simulink model "Ejercicio4_23_03_17"  (R2013a)
settings: Solver=ode45  StartTime=0.0  StopTime=10.0  RelTol=1e-3
libraries: powerlib x10, powerlib_meascontrol x3
settings Model: Creator=Miguel  LastModifiedBy=Miguel

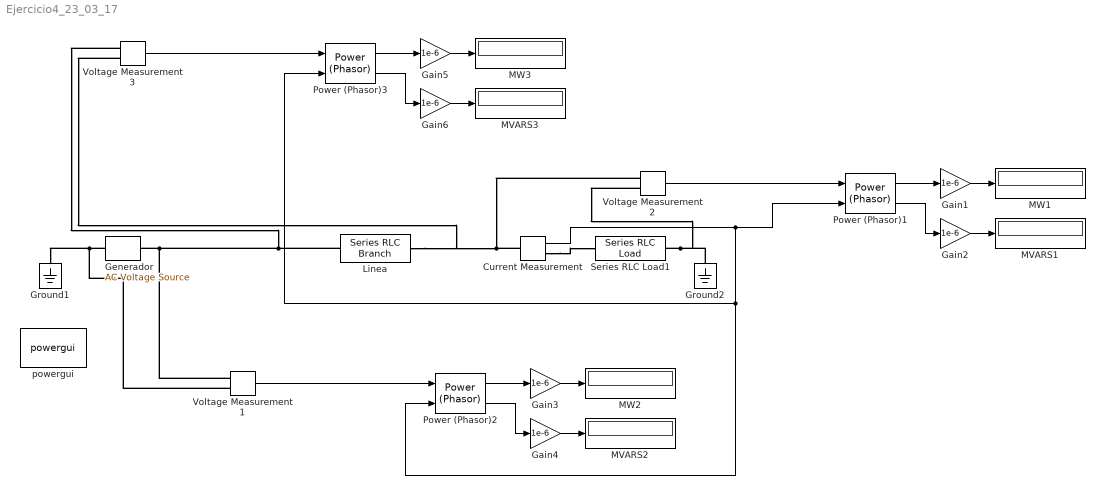
== system Ejercicio4_23_03_17 ==
  Current Measurement : powerlib/Measurements/Current Measurement  PhasorSimulation=on  OutputType=Complex  PSBequivalent=0
  Gain{1..6} (6 alike) : Gain  Gain=1e-6
  Generador : powerlib/Electrical Sources/AC Voltage Source  Amplitude=200e3*sqrt(2)  Phase=0  Frequency=60  SampleTime=0  Measurements=None
  Ground1 : powerlib/Elements/Ground  LConnTagsString=a
  Ground2 : powerlib/Elements/Ground  LConnTagsString=a
  Linea : powerlib/Elements/Series RLC Branch  LConnTagsString=__new0  RConnTagsString=__new0  BranchType=RL  Resistance=0.01*400  Inductance=0.1*400/(2*pi*60)  SetiL0=off  InitialCurrent=0  Capacitance=1e-6  Setx0=off  InitialVoltage=0  Measurements=None
  MVARS1 : Display
  MVARS2 : Display
  MVARS3 : Display
  MW1 : Display
  MW2 : Display
  MW3 : Display
  Power (Phasor)1 : powerlib_meascontrol/Measurements/Power (Phasor)
  Power (Phasor)2 : powerlib_meascontrol/Measurements/Power (Phasor)
  Power (Phasor)3 : powerlib_meascontrol/Measurements/Power (Phasor)
  Series RLC Load1 : powerlib/Elements/Series RLC Load  LConnTagsString=a  RConnTagsString=__new0  NominalVoltage=0.9624*200e3  NominalFrequency=60  ActivePower=0.5*100e6  InductivePower=0.3*100e6  CapacitivePower=0  Setx0=off  InitialVoltage=0  SetiL0=off  InitialCurrent=0  Measurements=None
  Voltage Measurement1 : powerlib/Measurements/Voltage Measurement  PhasorSimulation=on  OutputType=Complex  PSBequivalent=0
  Voltage Measurement2 : powerlib/Measurements/Voltage Measurement  PhasorSimulation=on  OutputType=Complex  PSBequivalent=0
  Voltage Measurement3 : powerlib/Measurements/Voltage Measurement  PhasorSimulation=on  OutputType=Complex  PSBequivalent=0
  powergui : powerlib/powergui  Priority=1  SimulationMode=Phasor  SolverType=Tustin  SampleTime=50e-6  frequency=60  SPID=off  DisableSnubberDevices=off  DisableRonSwitches=off  DisableVfSwitches=off  SwTol=0  Interpol=off  DisplayEquations=off  frequencyindice=60  Pbase=100e6  ErrMax=1e-4  Iterations=50  UnitsV=kV  UnitsW=MW  FunctionMessages=off  echomessages=off  HookPort=off  EnableUseOfTLC=off  x0status=blocks  RestoreLinks=warning  ResistiveCurrentMeasurement=off  Frange=[0:2:500]  Ylog=off  Xlog=on  ShowGrid=off  save=off  variable=ZData  ZoomFFT=off  StartTime=0.0  cycles=1  DisplayStyle=1  fundamental=60  FreqAxis=off  MaxFrequency=1000  frequencyindicesteady=1  RmsSteady=2  display=off  Ts=0  methode=off
  wires:
  Power (Phasor)1/1 -> Gain1/1
  Power (Phasor)1/2 -> Gain2/1
  Gain1/1 -> MW1/1
  Gain2/1 -> MVARS1/1
  Voltage Measurement2/1 -> Power (Phasor)1/1
  Power (Phasor)2/1 -> Gain3/1
  Power (Phasor)2/2 -> Gain4/1
  Gain3/1 -> MW2/1
  Gain4/1 -> MVARS2/1
  Current Measurement/1 -> Power (Phasor)3/2, Power (Phasor)2/2, Power (Phasor)1/2
  Voltage Measurement1/1 -> Power (Phasor)2/1
  Power (Phasor)3/1 -> Gain5/1
  Power (Phasor)3/2 -> Gain6/1
  Gain5/1 -> MW3/1
  Gain6/1 -> MVARS3/1
  Voltage Measurement3/1 -> Power (Phasor)3/1
  connections:
  Linea/LConn1 -- Voltage Measurement3/LConn1 -- Voltage Measurement1/LConn1 -- Generador/RConn1
  Voltage Measurement2/LConn1 -- Voltage Measurement3/LConn2 -- Linea/RConn1 -- Current Measurement/LConn1
  Series RLC Load1/RConn1 -- Ground2/LConn1 -- Voltage Measurement2/LConn2
  Current Measurement/RConn1 -- Series RLC Load1/LConn1
  Generador/LConn1 -- Voltage Measurement1/LConn2 -- Ground1/LConn1
